simulink model "intersampling_cl"  (R2023a)
settings: Solver=VariableStepAuto  StartTime=0.0  StopTime=10.0  RelTol=1e-3
libraries: simulink x1
settings Model: Creator=isaac  LastModifiedBy=isaac

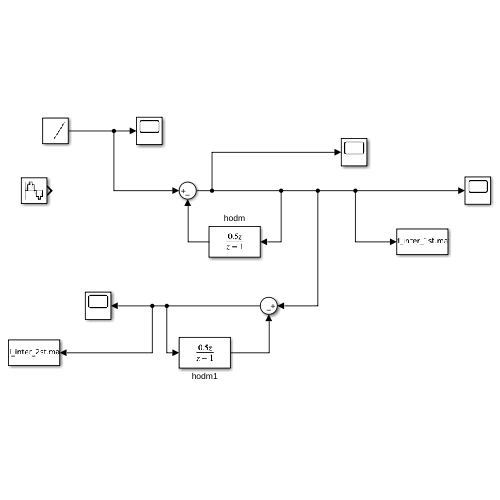
[thumbnail: Simulink's stored preview of the top-level diagram]
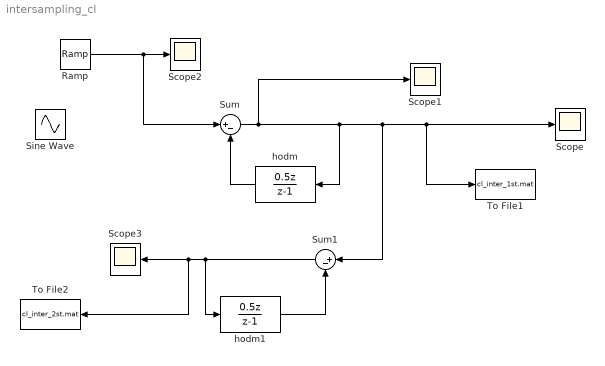
== system intersampling_cl ==
  Ramp : simulink/Sources/Ramp  slope=1  start=0  InitialOutput=0
  Scope{,1..3} (4 alike) : Scope
  Sine Wave : Sin  Frequency=80*pi  SampleTime=1/4000
  Sum : Sum  Inputs=|+-
  Sum1 : Sum  Inputs=|+-
  To File1 : ToFile  Filename=cl_inter_1st.mat  MatrixName=data  SampleTime=1/4000
  To File2 : ToFile  Filename=cl_inter_2st.mat  MatrixName=data  SampleTime=1/4000
  hodm : DiscreteTransferFcn  Numerator=[0.5 0]  Denominator=[1 -1]  SampleTime=1/1000
  hodm1 : DiscreteTransferFcn  Numerator=[0.5 0]  Denominator=[1 -1]  SampleTime=1/4000
  wires:
  Sum/1 -> Scope1/1, Sum1/1, To File1/1, Scope/1, hodm/1
  hodm/1 -> Sum/2
  Sum1/1 -> To File2/1, Scope3/1, hodm1/1
  hodm1/1 -> Sum1/2
  Ramp/1 -> Sum/1, Scope2/1
